simulink model "untitled"  (R2021b)
settings: Solver=VariableStepAuto  StartTime=0.0  StopTime=0.5  RelTol=1e-3
libraries: spsDCVoltageSourceLib x2, spsDCMachineLib x1, spspowerguiLib x1
settings Model: Creator=anacl  LastModifiedBy=anacl

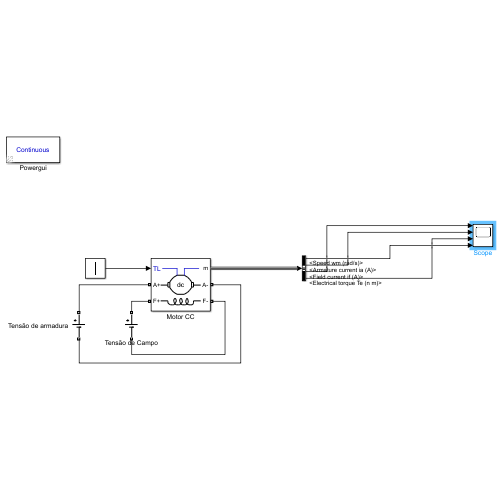
[thumbnail: Simulink's stored preview of the top-level diagram]
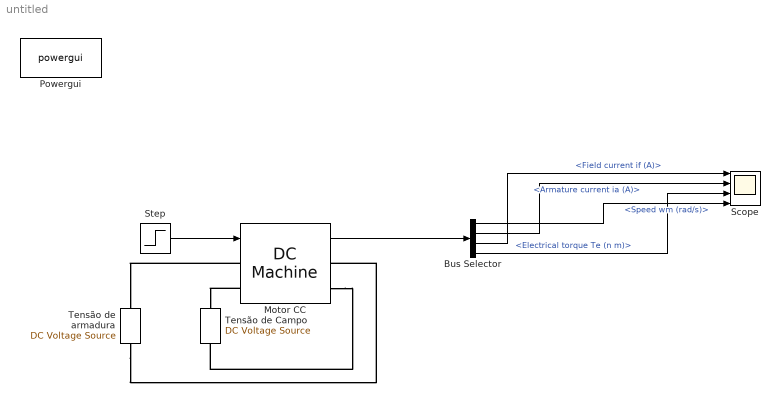
== system untitled ==
  Bus Selector : BusSelector  OutputSignals=Speed wm (rad/s),Armature current ia (A),Field current if (A),Electrical torque Te (n m)
  Motor CC : spsDCMachineLib/DC Machine  PresetModel=11: 40HP 500V 1750RPM Field:300V  MechanicalLoad=Torque TL  FieldType=Wound  ShowDetailedParameters=on  MeasurementBus=off  RLa=[0.6569 0.008734]  RLf=[92.78 16.23]  Laf=0.7688  MachineConstant=Torque constant (N.m/A)  Ke=1.8  Kt=1.8  J=0.1646  Bm=0.006126  Tf=4.223  w0=1  Ifinit=3.23345548609614  TsPowergui=0  TsBlock=-1
  Powergui : spspowerguiLib/powergui  Priority=1  SimulationMode=Continuous  SampleTime=50e-6  frequency=60  Iterations=50  frequencyindice=0  Pbase=100e6  ErrMax=1e-4  UnitsV=kV  UnitsW=MW  buscounter=0  FunctionMessages=off  echomessages=off  EnableUseOfTLC=off  CurrentSourceSwitches=off  DisableSnubberDevices=off  DisableRonSwitches=off  DisableVfSwitches=off  DisplayEquations=off  AutomaticDiscreteSolvers=off  SolverType=Tustin/Backward Euler (TBE)  Interpol=off  ExternalGateDelay=off  methode=off  Ts=100  x0status=blocks  SPID=on  SwTol=0  HookPort=off  NonlinearTolerance=1e-4  nMaxIteration=100  ContinueOnMaxIteration=off  RestoreLinks=warning  ResistiveCurrentMeasurement=off  Frange=[0:2:500]  Ylog=off  Xlog=on  ShowGrid=off  save=off  variable=ZData  structure=0  ZoomFFT=off  StartTime=0.0  cycles=1  DisplayStyle=1  fundamental=60  FreqAxis=off  MaxFrequency=1000  frequencyindicesteady=1  RmsSteady=1  display=off
  Scope : Scope  NumInputPorts=4
  Step : Step  After=81  SampleTime=0
  Tensão de Campo : spsDCVoltageSourceLib/DC Voltage Source  Amplitude=300  Measurements=None
  Tensão de armadura : spsDCVoltageSourceLib/DC Voltage Source  Amplitude=500  Measurements=None
  wires:
  Motor CC/1 -> Bus Selector/1
  Step/1 -> Motor CC/1
  Bus Selector/1 -> Scope/4  "<Speed wm (rad/s)>"
  Bus Selector/2 -> Scope/2  "<Armature current ia (A)>"
  Bus Selector/3 -> Scope/1  "<Field current if (A)>"
  Bus Selector/4 -> Scope/3  "<Electrical torque Te (n m)>"
  connections:
  Motor CC/LConn2 -- Tensão de Campo/RConn1
  Motor CC/RConn2 -- Tensão de Campo/LConn1
  Motor CC/LConn1 -- Tensão de armadura/RConn1
  Tensão de armadura/LConn1 -- Motor CC/RConn1
